simulink model "ABS_EV"  (R2020a)
settings: Solver=VariableStepAuto  StartTime=0.0  StopTime=12  RelTol=1e-3
undefined symbols (not defined in the file): g, I, m, R, v0
libraries: autolibshared x5, aerolibconvert2 x2
(part 3 of 3)

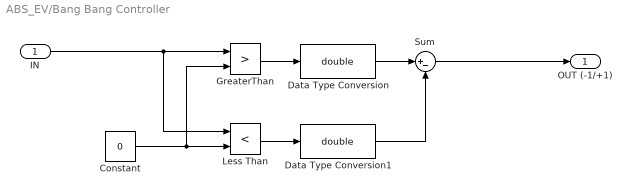
== system ABS_EV/Bang Bang Controller ==
  IN : Inport
  Constant : Constant  Value=0
  Data Type Conversion : DataTypeConversion  OutDataTypeStr=double  RndMeth=Zero
  Data Type Conversion1 : DataTypeConversion  OutDataTypeStr=double  RndMeth=Zero
  GreaterThan : RelationalOperator  Operator=>  OutDataTypeStr=boolean  RndMeth=Simplest
  Less Than : RelationalOperator  Operator=<  OutDataTypeStr=boolean  RndMeth=Simplest
  Sum : Sum  Inputs=|+-
  OUT (-1/+1) : Outport  VectorParamsAs1DForOutWhenUnconnected=off
  wires:
  Sum/1 -> OUT (-1/+1)/1
  Data Type Conversion/1 -> Sum/1
  Constant/1 -> GreaterThan/2, Less Than/2
  IN/1 -> Less Than/1, GreaterThan/1
  Data Type Conversion1/1 -> Sum/2
  GreaterThan/1 -> Data Type Conversion/1
  Less Than/1 -> Data Type Conversion1/1

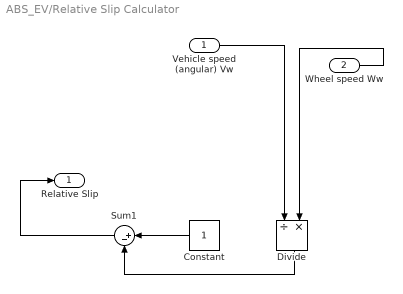
== system ABS_EV/Relative Slip Calculator ==
  Vehicle speed (angular) Vw : Inport
  Wheel speed Ww : Inport  Port=2
  Constant : Constant
  Divide : Product  Inputs=/*
  Sum1 : Sum  Inputs=|+-
  Relative Slip : Outport  VectorParamsAs1DForOutWhenUnconnected=off
  wires:
  Divide/1 -> Sum1/2
  Sum1/1 -> Relative Slip/1
  Constant/1 -> Sum1/1
  Wheel speed Ww/1 -> Divide/2
  Vehicle speed (angular) Vw/1 -> Divide/1

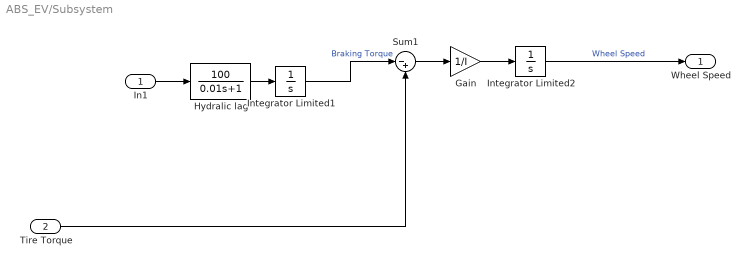
== system ABS_EV/Subsystem ==
  In1 : Inport
  Tire Torque : Inport  Port=2
  Gain : Gain  Gain=1/I
  Hydralic lag : TransferFcn  Numerator=[100]  Denominator=[0.01 1]
  Integrator Limited1 : Integrator  LimitOutput=on  UpperSaturationLimit=1500  LowerSaturationLimit=0
  Integrator Limited2 : Integrator  InitialCondition=v0/R  LimitOutput=on  UpperSaturationLimit=1000  LowerSaturationLimit=0
  Sum1 : Sum  Inputs=|-+
  Wheel Speed : Outport
  wires:
  Gain/1 -> Integrator Limited2/1
  Integrator Limited1/1 -> Sum1/1  "Braking Torque"
  Hydralic lag/1 -> Integrator Limited1/1
  Tire Torque/1 -> Sum1/2
  Sum1/1 -> Gain/1
  In1/1 -> Hydralic lag/1
  Integrator Limited2/1 -> Wheel Speed/1  "Wheel Speed"
